simulink model "lazo_abierto_a"  (R2021a)
settings: Solver=VariableStepAuto  StartTime=0.0  StopTime=500  RelTol=1e-3
values from neighbouring files (symbols this model uses):
  den = cell2mat(dem)    [Ajuste.m]    (also in Ajuste_COD.m = cell2mat(den))
settings Model: Creator=sebas  LastModifiedBy=sebas

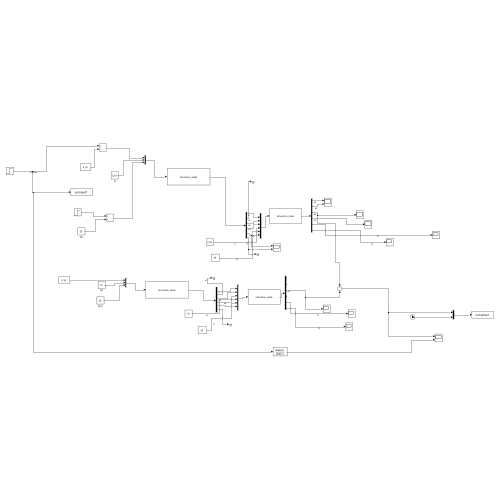
[thumbnail: Simulink's stored preview of the top-level diagram]
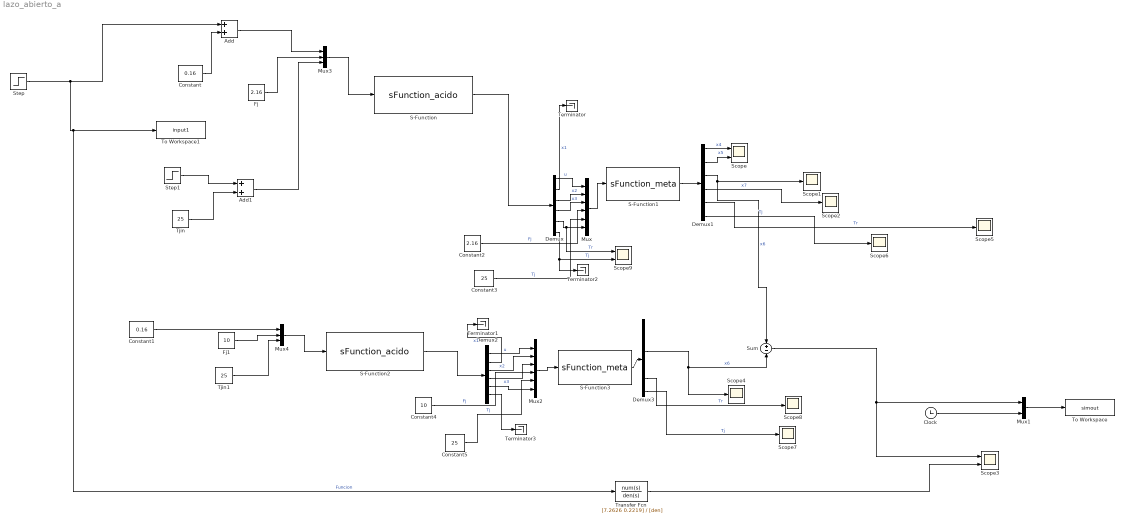
== system lazo_abierto_a ==
  Add : Sum
  Add1 : Sum
  Clock : Clock
  Constant : Constant  Value=0.16
  Constant1 : Constant  Value=0.16
  Constant2 : Constant  Value=2.16
  Constant3 : Constant  Value=25
  Constant4 : Constant  Value=10
  Constant5 : Constant  Value=25
  Demux{,1..3} (4 alike) : Demux  Outputs=6
  Fj : Constant  Value=2.16
  Fj1 : Constant  Value=10
  Mux : Mux  Inputs=6
  Mux1 : Mux  Inputs=2
  Mux2 : Mux  Inputs=6
  Mux3 : Mux  Inputs=3
  Mux4 : Mux  Inputs=3
  S-Function : S-Function  FunctionName=sFunction_acido  SFunctionDeploymentMode=off  EnableBusSupport=off
  S-Function1 : S-Function  FunctionName=sFunction_meta  SFunctionDeploymentMode=off  EnableBusSupport=off
  S-Function2 : S-Function  FunctionName=sFunction_acido  SFunctionDeploymentMode=off  EnableBusSupport=off
  S-Function3 : S-Function  FunctionName=sFunction_meta  SFunctionDeploymentMode=off  EnableBusSupport=off
  Scope : Scope  NumInputPorts=2
  Scope{1..2,4..8} (7 alike) : Scope
  Scope3 : Scope  NumInputPorts=2
  Scope9 : Scope  NumInputPorts=2
  Step : Step  Time=150  After=0.5*0.16  SampleTime=0
  Step1 : Step  Time=150  After=5  SampleTime=0
  Sum : Sum  Inputs=+-
  Terminator{,1..3} (4 alike) : Terminator
  Tjin : Constant  Value=25
  Tjin1 : Constant  Value=25
  To Workspace : ToWorkspace  VariableName=simout  SampleTime=0.1
  To Workspace1 : ToWorkspace  VariableName=input1  SampleTime=0.1
  Transfer Fcn : TransferFcn  Numerator=[7.2626 0.2219]  Denominator=[den]
  wires:
  Mux/1 -> S-Function1/1
  Demux1/4 -> Scope2/1  "x7"
  Demux1/3 -> Sum/1, Scope1/1  "x6"
  Demux1/2 -> Scope/2  "x5"
  Demux1/1 -> Scope/1  "x4"
  S-Function/1 -> Demux/1
  S-Function1/1 -> Demux1/1
  Constant/1 -> Add/2
  Add/1 -> Mux3/1
  Clock/1 -> Mux1/2
  Mux1/1 -> To Workspace/1
  Step/1 -> Transfer Fcn/1, To Workspace1/1, Add/1  "Funcion"
  Constant1/1 -> Mux4/1
  S-Function3/1 -> Demux3/1
  S-Function2/1 -> Demux2/1
  Mux2/1 -> S-Function3/1
  Demux3/3 -> Scope4/1, Sum/2  "x6"
  Sum/1 -> Mux1/1, Scope3/1
  Demux/1 -> Mux/1  "u"
  Demux/4 -> Mux/3  "x3"
  Demux/3 -> Mux/2  "x2"
  Demux/2 -> Terminator/1  "x1"
  Demux2/4 -> Mux2/3  "x3"
  Demux2/3 -> Mux2/2  "x2"
  Demux2/1 -> Mux2/1  "u"
  Demux2/2 -> Terminator1/1  "x1"
  Fj/1 -> Mux3/2
  Tjin/1 -> Add1/2
  Mux3/1 -> S-Function/1
  Demux/5 -> Scope9/1, Mux/6  "Tr"
  Demux/6 -> Terminator2/1, Scope9/2  "Tj"
  Constant2/1 -> Mux/4  "Fj"
  Constant3/1 -> Mux/5  "Tj"
  Demux1/5 -> Scope5/1  "Tr"
  Demux1/6 -> Scope6/1  "Tj"
  Tjin1/1 -> Mux4/3
  Fj1/1 -> Mux4/2
  Mux4/1 -> S-Function2/1
  Demux2/5 -> Mux2/6
  Demux2/6 -> Terminator3/1
  Constant4/1 -> Mux2/4  "Fj"
  Constant5/1 -> Mux2/5  "Tj"
  Demux3/6 -> Scope7/1  "Tj"
  Demux3/5 -> Scope8/1  "Tr"
  Step1/1 -> Add1/1
  Add1/1 -> Mux3/3
  Transfer Fcn/1 -> Scope3/2
